simulink model "SingleInverterSim"  (R2020b)
settings: Solver=FixedStepAuto  StartTime=0.0  StopTime=3  FixedStep=Ts  RelTol=1e-3
values from neighbouring files (symbols this model uses):
  Cf = 0.02/W    (= 6.36619772368e-05)    [CalcSwingDroop.m]    (also in SingleInverterSim_Para.m = 0.02; SingleInverterSim_Para_v2.m = 0.02)
  Lc = 0.01/W    (= 3.18309886184e-05)    [CalcSwingDroop.m]    (also in SingleInverterSim_Para.m = 1e-09; SingleInverterSim_Para_v2.m = 0.01)
  Lf = 0.05/W    (= 0.000159154943092)    [CalcSwingDroop.m]    (also in SingleInverterSim_Para.m = 0.05; SingleInverterSim_Para_v2.m = 0.05)
  m = m*Wbase    (= 15.7079632679)    [CalcSwingDroop.m]    (also in SingleInverterSim_Para.m = 0.05; SingleInverterSim_Para_v2.m = 0.05)
  R_rated_GFL = X_rated_GFL/5    (= 0.08)    [SingleInverterSim_Para.m]
  R_rated_GFM = X_rated_GFM/5    (= 0.06)    [SingleInverterSim_Para.m]
  Sbase = 1    [MainAnalysisImpedanceCircuit.m]    (also in SingleInverterSim_Para.m; SingleInverterSim_Para_v2.m)
  Scale_ki_v = 20    [SingleInverterSim_Para.m]    (also in SingleInverterSim_Para_v2.m)
  Ts = 1/Fs    (= 0.0001)    [SingleInverterSim_Para.m]    (also in SingleInverterSim_Para_v2.m)
  Vbase = 1    [MainAnalysisImpedanceCircuit.m]    (also in SingleInverterSim_Para.m; SingleInverterSim_Para_v2.m)
  w_droop = 0.1*2*pi    (= 0.628318530718)    [SingleInverterSim_Para.m]    (also in SingleInverterSim_Para_v2.m = 62.8318530718)
  w_i_GFL = 250 *2*pi    (= 1570.79632679)    [SingleInverterSim_Para.m]    (also in SingleInverterSim_Para_v2.m = 3141.59265359)
  w_i_GFM = 500*2*pi    (= 3141.59265359)    [SingleInverterSim_Para.m]    (also in SingleInverterSim_Para_v2.m)
  w_pll = 15 *2*pi    (= 94.2477796077)    [SingleInverterSim_Para.m]    (also in SingleInverterSim_Para_v2.m = 62.8318530718)
  w_tau = 1e3 *2*pi    (= 6283.18530718)    [SingleInverterSim_Para.m]    (also in SingleInverterSim_Para_v2.m)
  w_v_GFM = 250 *2*pi    (= 1570.79632679)    [SingleInverterSim_Para.m]    (also in SingleInverterSim_Para_v2.m)
  Wbase = 2*pi*50    (= 314.159265359)    [CalcSwingDroop.m]    (also in MainAnalysisImpedanceCircuit.m; SingleInverterSim_Para.m; SingleInverterSim_Para_v2.m)
  X_rated_GFL = 0.4    [SingleInverterSim_Para.m]
  X_rated_GFM = 0.3    [SingleInverterSim_Para.m]
  Zbase = Vbase/Ibase    (= 1)    [MainAnalysisImpedanceCircuit.m]    (also in SingleInverterSim_Para.m; SingleInverterSim_Para_v2.m)
undefined symbols (not defined in the file or in its folder): DiscIntNeverNeededParam, initial, magnitude
libraries: powerlib x230, SimplexPS x57, SimplexPS_2015a x10, SimplusGT x3
(part 3 of 5)

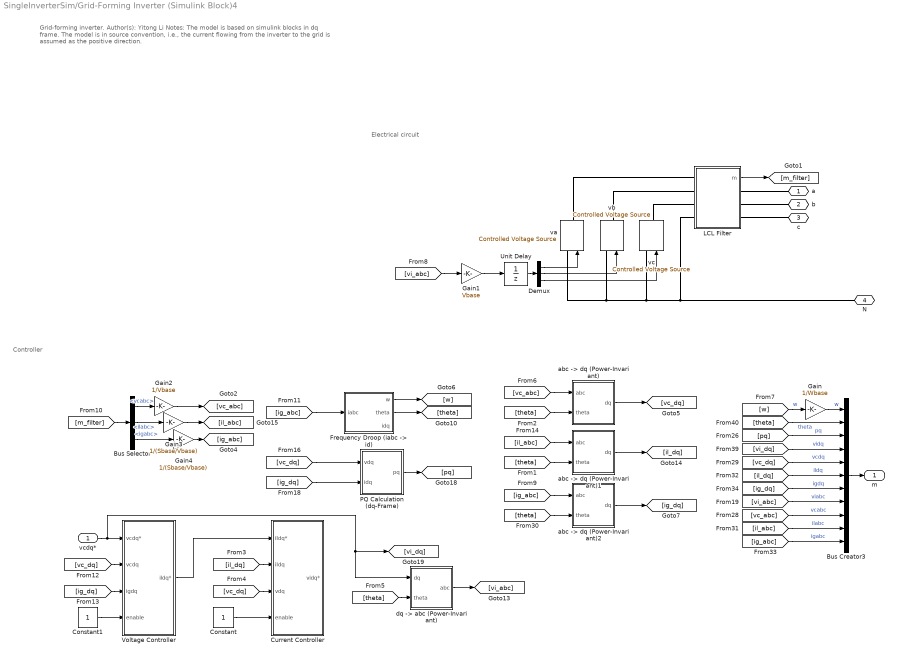
== system SingleInverterSim/Grid-Forming Inverter (Simulink Block)4 ==
  note: Grid-forming inverter.
      |
      | Author(s): Yitong Li
      |
      | Notes:
      |
      | The model is based on simulink blocks in dq frame.
      |
      | The model is in source convention, i.e., the current flowing from the inverter to the grid is assumed as the positive direction.
  note: Electrical circuit
  note: Controller
  vcdq* : Inport
  Bus Creator3 : BusCreator  Inputs=11
  Bus Selector : BusSelector  OutputSignals=vcabc,ilabc,igabc
  Constant : Constant
  Constant1 : Constant
  Current Controller : Subsystem  mask{Ts=Ts, Wbase=Wbase, Lf=Lf/Wbase, Kg=0, Kp=w_i*Lf/Wbase, Ki=w_i*w_i/4*Lf/Wbase, xdmax=inf, xqmax=inf, Kcd=0}
      mask prompts: Ts "Sampling Time (s)"; Wbase "Base Angular Frequency (rad/s)"; Lf "Inductance"; Kg "Estimator Gain"; Kp "Proportional Gain"; Ki "Integral Gain"; xdmax "Voltage D Limit"; xqmax "Voltage Q Limit"; Kcd "Cross Decoupling Gain"
  Demux : Demux  Outputs=3
  "Frequency Droop (iabc -> id)" : Subsystem  AncestorBlock=|  mask{Ts=Ts, Sbase=Sbase, Vbase=Vbase, Wbase=Wbase, m=m, w_tau=w_droop, theta0=0, i0=0, w0=1}
      | SimplusGT/Frequency Droop
      | (iabc -> id)
      mask prompts: Ts "Ts (s), samping period"; Sbase "Sbase (VA), base power"; Vbase "Vbase (V), base voltage"; Wbase "Wbase (rad/s), base angular frequency"; m "m (pu), droop gain"; w_tau "w_tau (rad/s), low-pass filter bandwidth"; theta0 "theta0 (rad), initial angle"; i0 "i0 (pu), current setting point"; w0 "w0 (pu), frequency setting point"
  Gain : Gain  Gain=1/Wbase
  Gain1 : Gain  Gain=Vbase
  Gain2 : Gain  Gain=1/Vbase
  Gain3 : Gain  Gain=1/(Sbase/Vbase)
  Gain4 : Gain  Gain=1/(Sbase/Vbase)
  LCL Filter : Subsystem  AncestorBlock=SimplexPS/LCL Filter  mask{Lf=Lf*(Vbase^2/Sbase)/Wbase, Rf=Lf*(Vbase^2/Sbase)/5, Lc=Lc*(Vbase^2/Sbase)/Wbase, Rc=Lc*(Vbase^2/Sbase)/5, Cf=Cf*(Sbase/Vbase^2)/Wbase, Rd=1e-5*(Vbase^2/Sbase)}
      mask prompts: Lf "Lf (H)"; Rf "Rf (Ohm)"; Lc "Lc (H)"; Rc "Rc (Ohm)"; Cf "Cf (F)"; Rd "Rd (Ohm)"
  PQ Calculation (dq-Frame) : Subsystem  AncestorBlock=|
      | SimplusGT/PQ Calculation
      | (dq-Frame)
  Unit Delay : UnitDelay  SampleTime=-1  HasFrameUpgradeWarning=on
  Voltage Controller : Subsystem  mask{Ts=Ts, Wbase=Wbase, Cf=Cf/Wbase, Kg=0, Kp=w_v*Cf/Wbase, Ki=w_v*w_v/4*Cf/Wbase*100, xdmax=inf, xqmax=inf, Kcd=0}
      mask prompts: Ts "Sampling Time (s)"; Wbase "Base Angular Frequency (rad/s)"; Cf "Capacitance"; Kg "Estimator Gain"; Kp "Proportional Gain"; Ki "Integral Gain"; xdmax "Current D Limit"; xqmax "Current Q Limit"; Kcd "Cross Decoupling Gain"
  "abc -> dq (Power-Invariant)" : Subsystem  AncestorBlock=|
      | SimplusGT/abc -> dq
      | (Power-Invariant)
  "abc -> dq (Power-Invariant)1" : Subsystem  AncestorBlock=|
      | SimplusGT/abc -> dq
      | (Power-Invariant)
  "abc -> dq (Power-Invariant)2" : Subsystem  AncestorBlock=|
      | SimplusGT/abc -> dq
      | (Power-Invariant)
  "dq -> abc (Power-Invariant)" : Subsystem  AncestorBlock=|
      | SimplusGT/dq -> abc
      | (Power-Invariant)
  va : powerlib/Electrical Sources/Controlled Voltage Source  Initialize=on  Source_Type=AC  Amplitude=0  Phase=0  Frequency=0  Measurements=None
  vb : powerlib/Electrical Sources/Controlled Voltage Source  Initialize=on  Source_Type=AC  Amplitude=0  Phase=0  Frequency=0  Measurements=None
  vc : powerlib/Electrical Sources/Controlled Voltage Source  Initialize=on  Source_Type=AC  Amplitude=0  Phase=0  Frequency=0  Measurements=None
  a : PMIOPort  Side=Right
  b : PMIOPort  Port=2  Side=Right
  c : PMIOPort  Port=3  Side=Right
  N : PMIOPort  Port=4  Side=Right
  m : Outport
  wires:
  Gain1/1 -> Unit Delay/1
  [vi_abc] -> Gain1/1
  Gain4/1 -> [ig_abc]
  Gain3/1 -> [il_abc]
  Gain2/1 -> [vc_abc]
  [ig_dq] -> Voltage Controller/3(igdq)
  [vc_dq] -> Voltage Controller/2(vcdq)
  Constant1/1 -> Voltage Controller/4(enable)
  Voltage Controller/1(ildq*) -> Current Controller/1(iIdq*)
  vcdq*/1 -> [vi_dq], "dq -> abc (Power-Invariant)"/1(dq), Voltage Controller/1(vcdq*)
  [ig_abc] -> Bus Creator3/11  "igabc"
  [il_abc] -> Bus Creator3/10  "ilabc"
  [vc_abc] -> Bus Creator3/9  "vcabc"
  [vi_abc] -> Bus Creator3/8  "viabc"
  [ig_dq] -> Bus Creator3/7  "igdq"
  [il_dq] -> Bus Creator3/6  "ildq"
  [vc_dq] -> Bus Creator3/5  "vcdq"
  [vi_dq] -> Bus Creator3/4  "vidq"
  [pq] -> Bus Creator3/3  "pq"
  [theta] -> Bus Creator3/2  "theta"
  Gain/1 -> Bus Creator3/1  "w"
  [w] -> Gain/1  "w"
  Bus Selector/1 -> Gain2/1  "<vcabc>"
  Unit Delay/1 -> Demux/1
  [m_filter] -> Bus Selector/1
  "abc -> dq (Power-Invariant)1"/1(dq) -> [il_dq]
  "abc -> dq (Power-Invariant)2"/1(dq) -> [ig_dq]
  "abc -> dq (Power-Invariant)"/1(dq) -> [vc_dq]
  [ig_abc] -> "Frequency Droop (iabc -> id)"/1(iabc)
  [il_dq] -> Current Controller/2(iIdq)
  [ig_dq] -> PQ Calculation (dq-Frame)/2(idq)
  PQ Calculation (dq-Frame)/1(pq) -> [pq]
  [vc_dq] -> PQ Calculation (dq-Frame)/1(vdq)
  [theta] -> "dq -> abc (Power-Invariant)"/2(theta)
  [vc_dq] -> Current Controller/3(vdq)
  Constant/1 -> Current Controller/4(enable)
  Bus Selector/2 -> Gain3/1  "<ilabc>"
  Bus Selector/3 -> Gain4/1  "<igabc>"
  [theta] -> "abc -> dq (Power-Invariant)2"/2(theta)
  [ig_abc] -> "abc -> dq (Power-Invariant)2"/1(abc)
  [il_abc] -> "abc -> dq (Power-Invariant)1"/1(abc)
  [vc_abc] -> "abc -> dq (Power-Invariant)"/1(abc)
  [theta] -> "abc -> dq (Power-Invariant)1"/2(theta)
  [theta] -> "abc -> dq (Power-Invariant)"/2(theta)
  Demux/3 -> vc/1
  Demux/2 -> vb/1
  Demux/1 -> va/1
  LCL Filter/1(m) -> [m_filter]
  Bus Creator3/1 -> m/1
  "dq -> abc (Power-Invariant)"/1(abc) -> [vi_abc]
  "Frequency Droop (iabc -> id)"/1(w) -> [w]
  "Frequency Droop (iabc -> id)"/2(theta) -> [theta]
  connections:
  LCL Filter/LConn3 -- vc/RConn1
  va/LConn1 -- vb/LConn1 -- vc/LConn1 -- LCL Filter/LConn4 -- N/RConn1
  LCL Filter/RConn3 -- c/RConn1
  LCL Filter/RConn2 -- b/RConn1
  LCL Filter/RConn1 -- a/RConn1
  LCL Filter/LConn1 -- va/RConn1
  LCL Filter/LConn2 -- vb/RConn1

== system SingleInverterSim/Grid-Following Inverter (Simulink Block)1/Current Controller ==
  iIdq* : Inport
  iIdq : Inport  Port=2
  vdq : Inport  Port=3
  enable : Inport  Port=4
  Constant : Constant  Value=Kcd
  Demux1 : Demux  Outputs=2
  Demux2 : Demux  Outputs=2
  Demux3 : Demux  Outputs=2
  Mux : Mux  Inputs=2
  PI-DT-Estimated d : Subsystem  mask{Lf=Lf, Kg=Kg, Kp=Kp, Ki=Ki, xmax=vdmax, xmin=-vdmax, Ts=Ts}
      mask prompts: Lf "Inductance"; Kg "Estimator Gain"; Kp "Proportional Gain"; Ki "Integral Gain"; xmax "Upper Limit"; xmin "Lower Limit"; Ts "Sampling Time"
  PI-DT-Estimated q : Subsystem  mask{Lf=Lf, Kg=Kg, Kp=Kp, Ki=Ki, xmax=vqmax, xmin=-vqmax, Ts=Ts}
      mask prompts: Lf "Inductance"; Kg "Estimator Gain"; Kp "Proportional Gain"; Ki "Integral Gain"; xmax "Upper Limit"; xmin "Lower Limit"; Ts "Sampling Time"
  Product : Product
  Product1 : Product
  sum_d : Sum  Inputs=+-
  sum_q : Sum
  wLd : Gain  Gain=Wbase*Lf
  wLq : Gain  Gain=Wbase*Lf
  vidq* : Outport
  wires:
  Constant/1 -> Product1/1, Product/2
  Product1/1 -> sum_d/2
  wLq/1 -> Product1/2
  Product/1 -> sum_q/1
  wLd/1 -> Product/1
  enable/1 -> PI-DT-Estimated d/1(enable), PI-DT-Estimated q/4(enable)
  Demux2/2 -> PI-DT-Estimated q/3(reference)
  Demux2/1 -> PI-DT-Estimated d/2(reference)
  iIdq*/1 -> Demux2/1
  Demux3/1 -> PI-DT-Estimated d/3(initial)
  Demux3/2 -> PI-DT-Estimated q/2(initial)
  PI-DT-Estimated q/1(Out) -> sum_q/2
  vdq/1 -> Demux3/1
  PI-DT-Estimated d/1(Out) -> sum_d/1
  Mux/1 -> vidq*/1
  Demux1/2 -> wLq/1, PI-DT-Estimated q/1(actual)
  Demux1/1 -> PI-DT-Estimated d/4(actual), wLd/1
  iIdq/1 -> Demux1/1
  sum_q/1 -> Mux/2
  sum_d/1 -> Mux/1

== system SingleInverterSim/Grid-Following Inverter (Simulink Block)1/LCL Filter ==
  note: Model for a LCL filter.
      |
      | Author(s): Yitong Li
      |
      | Notes:
      |
      | vi is the converter side voltage, and vg is the grid side voltage.
  Bus Creator : BusCreator  Inputs=5
  "LL -> LN1" : Subsystem  AncestorBlock=|
      | SimplusGT/Grid-Forming Inverter
      | (Simulink Block)/LCL Filter/LL -> LN1
  "LL -> LN2" : Subsystem  AncestorBlock=|
      | SimplusGT/Grid-Forming Inverter
      | (Simulink Block)/LCL Filter/LL -> LN1
  Mux{,1..4} (5 alike) : Mux  Inputs=3
  Three-Phase Series RLC Branch : powerlib/Elements/Three-Phase Series RLC Branch  LConnTagsString=A|B|C  RConnTagsString=A|B|C  BranchType=RL  Resistance=Rf  Inductance=Lf  Capacitance=1e-6  Measurements=None
  Three-Phase Series RLC Branch1 : powerlib/Elements/Three-Phase Series RLC Branch  LConnTagsString=A|B|C  RConnTagsString=A|B|C  BranchType=RL  Resistance=Rc  Inductance=Lc  Capacitance=1e-6  Measurements=None
  Three-Phase Series RLC Branch2 : powerlib/Elements/Three-Phase Series RLC Branch  LConnTagsString=A|B|C  RConnTagsString=A|B|C  BranchType=RC  Resistance=Rd  Inductance=Lc  Capacitance=Cf  Measurements=None
  Vab : powerlib/Measurements/Voltage Measurement  PhasorSimulation=off  OutputType=Complex  PSBequivalent=0
  Vab1 : powerlib/Measurements/Voltage Measurement  PhasorSimulation=off  OutputType=Complex  PSBequivalent=0
  Vbc : powerlib/Measurements/Voltage Measurement  PhasorSimulation=off  OutputType=Complex  PSBequivalent=0
  Vbc1 : powerlib/Measurements/Voltage Measurement  PhasorSimulation=off  OutputType=Complex  PSBequivalent=0
  Vca : powerlib/Measurements/Voltage Measurement  PhasorSimulation=off  OutputType=Complex  PSBequivalent=0
  Vca1 : powerlib/Measurements/Voltage Measurement  PhasorSimulation=off  OutputType=Complex  PSBequivalent=0
  iga : powerlib/Measurements/Current Measurement  PhasorSimulation=off  OutputType=Complex  PSBequivalent=0
  igb : powerlib/Measurements/Current Measurement  PhasorSimulation=off  OutputType=Complex  PSBequivalent=0
  igc : powerlib/Measurements/Current Measurement  PhasorSimulation=off  OutputType=Complex  PSBequivalent=0
  ila : powerlib/Measurements/Current Measurement  PhasorSimulation=off  OutputType=Complex  PSBequivalent=0
  ilb : powerlib/Measurements/Current Measurement  PhasorSimulation=off  OutputType=Complex  PSBequivalent=0
  ilc : powerlib/Measurements/Current Measurement  PhasorSimulation=off  OutputType=Complex  PSBequivalent=0
  vca measure : powerlib/Measurements/Voltage Measurement  PhasorSimulation=off  OutputType=Complex  PSBequivalent=0
  vcb measure : powerlib/Measurements/Voltage Measurement  PhasorSimulation=off  OutputType=Complex  PSBequivalent=0
  vcc measure : powerlib/Measurements/Voltage Measurement  PhasorSimulation=off  OutputType=Complex  PSBequivalent=0
  via : PMIOPort  Side=Left
  vib : PMIOPort  Port=2  Side=Left
  vic : PMIOPort  Port=3  Side=Left
  vga : PMIOPort  Port=4  Side=Right
  vgb : PMIOPort  Port=5  Side=Right
  vgc : PMIOPort  Port=6  Side=Right
  N : PMIOPort  Port=7  Side=Left
  m : Outport
  wires:
  Mux4/1 -> [igabc]
  ilb/1 -> Mux2/2
  ila/1 -> Mux2/1
  igc/1 -> Mux4/3
  vcc measure/1 -> Mux3/3
  Vab/1 -> Mux/1
  Mux/1 -> "LL -> LN1"/1(In1)
  vca measure/1 -> Mux3/1
  vcb measure/1 -> Mux3/2
  igb/1 -> Mux4/2
  iga/1 -> Mux4/1
  Vca/1 -> Mux/3
  ilc/1 -> Mux2/3
  Vbc/1 -> Mux/2
  Mux2/1 -> [ilabc]
  Bus Creator/1 -> m/1
  "LL -> LN1"/1(Out1) -> [vgabc]
  Mux3/1 -> [vcabc]
  Vbc1/1 -> Mux1/2
  Vca1/1 -> Mux1/3
  Mux1/1 -> "LL -> LN2"/1(In1)
  Vab1/1 -> Mux1/1
  "LL -> LN2"/1(Out1) -> [viabc]
  [viabc] -> Bus Creator/1  "viabc"
  [vcabc] -> Bus Creator/2  "vcabc"
  [vgabc] -> Bus Creator/3  "vgabc"
  [ilabc] -> Bus Creator/4  "ilabc"
  [igabc] -> Bus Creator/5  "igabc"
  connections:
  Three-Phase Series RLC Branch2/RConn1 -- Three-Phase Series RLC Branch2/RConn2 -- N/RConn1 -- Three-Phase Series RLC Branch2/RConn3 -- vcc measure/LConn2 -- vca measure/LConn2 -- vcb measure/LConn2
  Vca/LConn1 -- Vbc/LConn2 -- igc/RConn1 -- vgc/RConn1
  Vca1/LConn1 -- Vbc1/LConn2 -- vic/RConn1 -- Three-Phase Series RLC Branch/LConn3
  Three-Phase Series RLC Branch/LConn2 -- Vbc1/LConn1 -- Vab1/LConn2 -- vib/RConn1
  Vab1/LConn1 -- Vca1/LConn2 -- via/RConn1 -- Three-Phase Series RLC Branch/LConn1
  Three-Phase Series RLC Branch1/LConn3 -- ilc/RConn1 -- Three-Phase Series RLC Branch2/LConn3 -- vcc measure/LConn1
  Three-Phase Series RLC Branch1/RConn2 -- igb/LConn1
  Vbc/LConn1 -- Vab/LConn2 -- igb/RConn1 -- vgb/RConn1
  ilb/RConn1 -- Three-Phase Series RLC Branch1/LConn2 -- vcb measure/LConn1 -- Three-Phase Series RLC Branch2/LConn2
  ila/RConn1 -- Three-Phase Series RLC Branch1/LConn1 -- vca measure/LConn1 -- Three-Phase Series RLC Branch2/LConn1
  Vab/LConn1 -- Vca/LConn2 -- iga/RConn1 -- vga/RConn1
  Three-Phase Series RLC Branch1/RConn1 -- iga/LConn1
  Three-Phase Series RLC Branch1/RConn3 -- igc/LConn1
  Three-Phase Series RLC Branch/RConn1 -- ila/LConn1
  Three-Phase Series RLC Branch/RConn2 -- ilb/LConn1
  Three-Phase Series RLC Branch/RConn3 -- ilc/LConn1

== system SingleInverterSim/Grid-Following Inverter (Simulink Block)1/PLL (vabc -> vq) ==
  note: Measurement
  note: Gpll
  note: Phase lock loop (PLL)
      |
      | Author(s): Yitong Li
      |
      | Notes:
      |
      | vq is fed into the PI controller of the PLL.
  vabc : Inport
  Constant1 : Constant
  Constant2 : Constant  Value=theta0
  Constant3 : Constant
  Constant4 : Constant  Value=2*pi
  Constant6 : Constant  Value=0
  Demux1 : Demux  Outputs=2
  Discrete PI : Subsystem  AncestorBlock=SimplusGT/Discrete PI  mask{Kp=w_pll, Ki=w_pll*w_pll/4, xmax=inf, xmin=-inf, Ts=Ts}
      mask prompts: Kp "Proportional Gain"; Ki "Integral Gain"; xmax "Upper Limit"; xmin "Lower Limit"; Ts "Sampling Time"
  Discrete-Time Integrator : DiscreteIntegrator  SampleTime=Ts  ICPrevOutput=DiscIntNeverNeededParam  ICPrevScaledInput=DiscIntNeverNeededParam
  Filter p : DiscreteTransferFcn  Commented=on  Numerator=w_tau*Ts  Denominator=[1 ((w_tau*Ts)-1)]  SampleTime=Ts
  Gain1 : Gain  Gain=Wbase
  Gain4 : Gain  Gain=1/Wbase
  Gain5 : Gain  Gain=1/pi
  Math Function1 : Math  Operator=mod  SignedPower=on  SaturateOnIntegerOverflow=on
  Mux : Mux  Inputs=2
  Scope : Scope  NumInputPorts=4
  Sum : Sum
  Sum1 : Sum
  "abc -> dq (Power-Invariant)" : Subsystem  AncestorBlock=|
      | SimplusGT/abc -> dq
      | (Power-Invariant)
  w : Outport
  theta : Outport  Port=2
  vdq : Outport  Port=3
  wires:
  vabc/1 -> "abc -> dq (Power-Invariant)"/1(abc)
  "abc -> dq (Power-Invariant)"/1(dq) -> vdq/1, Demux1/1
  Constant4/1 -> Math Function1/2
  Constant6/1 -> Discrete PI/4(actual), Discrete PI/3(initial)
  Constant1/1 -> Discrete PI/1(enable)
  Discrete PI/1(Out) -> Sum/1
  Sum/1 -> [w], w/1, Discrete-Time Integrator/1
  Gain1/1 -> Sum/2
  Discrete-Time Integrator/1 -> Sum1/1
  Sum1/1 -> Math Function1/1
  Constant2/1 -> [theta0], Sum1/2
  Demux1/2 -> Discrete PI/2(reference), [vq]
  [vq] -> Scope/2  "vq"
  Mux/1 -> Gain5/1
  Gain4/1 -> Scope/3
  [w] -> Gain4/1  "w"
  [theta0] -> Mux/1  "theta0"
  [vd] -> Scope/1  "vd"
  Gain5/1 -> Scope/4
  [theta] -> Mux/2  "theta"
  Demux1/1 -> [vd]
  Constant3/1 -> Gain1/1
  Math Function1/1 -> "abc -> dq (Power-Invariant)"/2(theta), [theta], theta/1

== system SingleInverterSim/Grid-Following Inverter (Simulink Block)1/PQ Calculation (dq-Frame)1 ==
  note: Power calculation.
      |
      | Author(s): Yitong Li
      |
      | Notes:
      |
      | The calculation is done in dq frame.
  vdq : Inport
  idq : Inport  Port=2
  Mux : Mux  Inputs=2
  Mux1 : Mux  Inputs=2
  P = vd*id+vq*iq : Fcn  Expr=u[1]*u[3]+u[2]*u[4]
  Q = -vd*iq+vq*id : Fcn  Expr=-u[1]*u[4]+u[2]*u[3]
  pq : Outport
  wires:
  Mux/1 -> pq/1
  P = vd*id+vq*iq/1 -> Mux/1
  vdq/1 -> Mux1/1
  idq/1 -> Mux1/2
  Mux1/1 -> P = vd*id+vq*iq/1, Q = -vd*iq+vq*id/1
  Q = -vd*iq+vq*id/1 -> Mux/2

== system SingleInverterSim/Grid-Following Inverter (Simulink Block)1/abc -> dq (Power-Invariant)1 ==
  note: Frame transformation from abc to dq.
      |
      | Author(s): Yitong Li
      |
      | Notes:
      |
      | The transformation is power-invariant.
      |
      | theta is the angle that d axis leads a axis.
      |
      | q axis leads d axis by 90 degrees.
  abc : Inport
  theta : Inport  Port=2
  ->d : Fcn  Expr=cos(u(4))*u(1) + cos(u(4)-2/3*pi)*u(2) + cos(u(4)-4/3*pi)*u(3)
  ->q : Fcn  Expr=-sin(u(4))*u(1) - sin(u(4)-2/3*pi)*u(2) - sin(u(4)-4/3*pi)*u(3)
  Gain : Gain  Gain=sqrt(2/3)
  Mux5 : Mux  Inputs=2
  Mux6 : Mux  Inputs=2
  dq : Outport
  wires:
  abc/1 -> Gain/1
  ->d/1 -> Mux6/1
  Gain/1 -> Mux5/1
  theta/1 -> Mux5/2
  ->q/1 -> Mux6/2
  Mux6/1 -> dq/1
  Mux5/1 -> ->d/1, ->q/1

== system SingleInverterSim/Grid-Following Inverter (Simulink Block)1/abc -> dq (Power-Invariant)2 ==
  note: Frame transformation from abc to dq.
      |
      | Author(s): Yitong Li
      |
      | Notes:
      |
      | The transformation is power-invariant.
      |
      | theta is the angle that d axis leads a axis.
      |
      | q axis leads d axis by 90 degrees.
  abc : Inport
  theta : Inport  Port=2
  ->d : Fcn  Expr=cos(u(4))*u(1) + cos(u(4)-2/3*pi)*u(2) + cos(u(4)-4/3*pi)*u(3)
  ->q : Fcn  Expr=-sin(u(4))*u(1) - sin(u(4)-2/3*pi)*u(2) - sin(u(4)-4/3*pi)*u(3)
  Gain : Gain  Gain=sqrt(2/3)
  Mux5 : Mux  Inputs=2
  Mux6 : Mux  Inputs=2
  dq : Outport
  wires:
  abc/1 -> Gain/1
  ->d/1 -> Mux6/1
  Gain/1 -> Mux5/1
  theta/1 -> Mux5/2
  ->q/1 -> Mux6/2
  Mux6/1 -> dq/1
  Mux5/1 -> ->d/1, ->q/1

== system SingleInverterSim/Grid-Following Inverter (Simulink Block)1/abc -> dq (Power-Invariant)4 ==
  note: Frame transformation from abc to dq.
      |
      | Author(s): Yitong Li
      |
      | Notes:
      |
      | The transformation is power-invariant.
      |
      | theta is the angle that d axis leads a axis.
      |
      | q axis leads d axis by 90 degrees.
  abc : Inport
  theta : Inport  Port=2
  ->d : Fcn  Expr=cos(u(4))*u(1) + cos(u(4)-2/3*pi)*u(2) + cos(u(4)-4/3*pi)*u(3)
  ->q : Fcn  Expr=-sin(u(4))*u(1) - sin(u(4)-2/3*pi)*u(2) - sin(u(4)-4/3*pi)*u(3)
  Gain : Gain  Gain=sqrt(2/3)
  Mux5 : Mux  Inputs=2
  Mux6 : Mux  Inputs=2
  dq : Outport
  wires:
  abc/1 -> Gain/1
  ->d/1 -> Mux6/1
  Gain/1 -> Mux5/1
  theta/1 -> Mux5/2
  ->q/1 -> Mux6/2
  Mux6/1 -> dq/1
  Mux5/1 -> ->d/1, ->q/1

== system SingleInverterSim/Grid-Following Inverter (Simulink Block)1/dq -> abc (Power-Invariant)1 ==
  note: Frame transformation from dq to abc.
      |
      | Author(s): Yitong Li
      |
      | Notes:
      |
      | The transformation is power-invariant.
      |
      | theta is the angle that dq axis leads alpha/beta axis, specifically, d axis leads alpha axis.
  dq : Inport
  theta : Inport  Port=2
  ->a : Fcn  Expr=cos(u(3))*u(1) - sin(u(3))*u(2)
  ->b : Fcn  Expr=cos(u(3)-2/3*pi)*u(1) - sin(u(3)-2/3*pi)*u(2)
  ->c : Fcn  Expr=cos(u(3)-4/3*pi)*u(1) - sin(u(3)-4/3*pi)*u(2)
  Gain : Gain  Gain=sqrt(2/3)
  Mux5 : Mux  Inputs=2
  Mux6 : Mux  Inputs=3
  abc : Outport
  wires:
  ->b/1 -> Mux6/2
  ->a/1 -> Mux6/1
  Gain/1 -> Mux5/1
  dq/1 -> Gain/1
  ->c/1 -> Mux6/3
  Mux6/1 -> abc/1
  Mux5/1 -> ->b/1, ->a/1, ->c/1
  theta/1 -> Mux5/2

== system SingleInverterSim/Grid-Following Inverter (Simulink Block)2/Current Controller ==
  iIdq* : Inport
  iIdq : Inport  Port=2
  vdq : Inport  Port=3
  enable : Inport  Port=4
  Constant : Constant  Value=Kcd
  Demux1 : Demux  Outputs=2
  Demux2 : Demux  Outputs=2
  Demux3 : Demux  Outputs=2
  Mux : Mux  Inputs=2
  PI-DT-Estimated d : Subsystem  mask{Lf=Lf, Kg=Kg, Kp=Kp, Ki=Ki, xmax=vdmax, xmin=-vdmax, Ts=Ts}
      mask prompts: Lf "Inductance"; Kg "Estimator Gain"; Kp "Proportional Gain"; Ki "Integral Gain"; xmax "Upper Limit"; xmin "Lower Limit"; Ts "Sampling Time"
  PI-DT-Estimated q : Subsystem  mask{Lf=Lf, Kg=Kg, Kp=Kp, Ki=Ki, xmax=vqmax, xmin=-vqmax, Ts=Ts}
      mask prompts: Lf "Inductance"; Kg "Estimator Gain"; Kp "Proportional Gain"; Ki "Integral Gain"; xmax "Upper Limit"; xmin "Lower Limit"; Ts "Sampling Time"
  Product : Product
  Product1 : Product
  sum_d : Sum  Inputs=+-
  sum_q : Sum
  wLd : Gain  Gain=Wbase*Lf
  wLq : Gain  Gain=Wbase*Lf
  vidq* : Outport
  wires:
  sum_d/1 -> Mux/1
  sum_q/1 -> Mux/2
  iIdq/1 -> Demux1/1
  Demux1/1 -> wLd/1, PI-DT-Estimated d/4(actual)
  Demux1/2 -> PI-DT-Estimated q/1(actual), wLq/1
  Mux/1 -> vidq*/1
  PI-DT-Estimated d/1(Out) -> sum_d/1
  vdq/1 -> Demux3/1
  PI-DT-Estimated q/1(Out) -> sum_q/2
  Demux3/2 -> PI-DT-Estimated q/2(initial)
  Demux3/1 -> PI-DT-Estimated d/3(initial)
  iIdq*/1 -> Demux2/1
  Demux2/1 -> PI-DT-Estimated d/2(reference)
  Demux2/2 -> PI-DT-Estimated q/3(reference)
  enable/1 -> PI-DT-Estimated q/4(enable), PI-DT-Estimated d/1(enable)
  wLd/1 -> Product/1
  Product/1 -> sum_q/1
  wLq/1 -> Product1/2
  Product1/1 -> sum_d/2
  Constant/1 -> Product/2, Product1/1

== system SingleInverterSim/Grid-Following Inverter (Simulink Block)2/LCL Filter ==
  note: Model for a LCL filter.
      |
      | Author(s): Yitong Li
      |
      | Notes:
      |
      | vi is the converter side voltage, and vg is the grid side voltage.
  Bus Creator : BusCreator  Inputs=5
  "LL -> LN" : SimplexPS_2015a/LL -> LN  SystemSampleTime=-1  VariantActivationTime=update diagram  Latency=0  AutoFrameSizeCalculation=off
  "LL -> LN1" : SimplexPS_2015a/LL -> LN  SystemSampleTime=-1  VariantActivationTime=update diagram  Latency=0  AutoFrameSizeCalculation=off
  Mux{,1..4} (5 alike) : Mux  Inputs=3
  Three-Phase Series RLC Branch : powerlib/Elements/Three-Phase Series RLC Branch  LConnTagsString=A|B|C  RConnTagsString=A|B|C  BranchType=RL  Resistance=Rf  Inductance=Lf  Capacitance=1e-6  Measurements=None
  Three-Phase Series RLC Branch1 : powerlib/Elements/Three-Phase Series RLC Branch  LConnTagsString=A|B|C  RConnTagsString=A|B|C  BranchType=RL  Resistance=Rc  Inductance=Lc  Capacitance=1e-6  Measurements=None
  Three-Phase Series RLC Branch2 : powerlib/Elements/Three-Phase Series RLC Branch  LConnTagsString=A|B|C  RConnTagsString=A|B|C  BranchType=RC  Resistance=Rd  Inductance=Lc  Capacitance=Cf  Measurements=None
  Vab : powerlib/Measurements/Voltage Measurement  PhasorSimulation=off  OutputType=Complex  PSBequivalent=0
  Vab1 : powerlib/Measurements/Voltage Measurement  PhasorSimulation=off  OutputType=Complex  PSBequivalent=0
  Vbc : powerlib/Measurements/Voltage Measurement  PhasorSimulation=off  OutputType=Complex  PSBequivalent=0
  Vbc1 : powerlib/Measurements/Voltage Measurement  PhasorSimulation=off  OutputType=Complex  PSBequivalent=0
  Vca : powerlib/Measurements/Voltage Measurement  PhasorSimulation=off  OutputType=Complex  PSBequivalent=0
  Vca1 : powerlib/Measurements/Voltage Measurement  PhasorSimulation=off  OutputType=Complex  PSBequivalent=0
  iga : powerlib/Measurements/Current Measurement  PhasorSimulation=off  OutputType=Complex  PSBequivalent=0
  igb : powerlib/Measurements/Current Measurement  PhasorSimulation=off  OutputType=Complex  PSBequivalent=0
  igc : powerlib/Measurements/Current Measurement  PhasorSimulation=off  OutputType=Complex  PSBequivalent=0
  ila : powerlib/Measurements/Current Measurement  PhasorSimulation=off  OutputType=Complex  PSBequivalent=0
  ilb : powerlib/Measurements/Current Measurement  PhasorSimulation=off  OutputType=Complex  PSBequivalent=0
  ilc : powerlib/Measurements/Current Measurement  PhasorSimulation=off  OutputType=Complex  PSBequivalent=0
  vca measure : powerlib/Measurements/Voltage Measurement  PhasorSimulation=off  OutputType=Complex  PSBequivalent=0
  vcb measure : powerlib/Measurements/Voltage Measurement  PhasorSimulation=off  OutputType=Complex  PSBequivalent=0
  vcc measure : powerlib/Measurements/Voltage Measurement  PhasorSimulation=off  OutputType=Complex  PSBequivalent=0
  via : PMIOPort  Side=Left
  vib : PMIOPort  Port=2  Side=Left
  vic : PMIOPort  Port=3  Side=Left
  vga : PMIOPort  Port=4  Side=Right
  vgb : PMIOPort  Port=5  Side=Right
  vgc : PMIOPort  Port=6  Side=Right
  N : PMIOPort  Port=7  Side=Left
  m : Outport
  wires:
  [igabc] -> Bus Creator/5  "igabc"
  [ilabc] -> Bus Creator/4  "ilabc"
  [vgabc] -> Bus Creator/3  "vgabc"
  [vcabc] -> Bus Creator/2  "vcabc"
  [viabc] -> Bus Creator/1  "viabc"
  "LL -> LN"/1 -> [viabc]
  Vab1/1 -> Mux1/1
  Mux1/1 -> "LL -> LN"/1
  Vca1/1 -> Mux1/3
  Vbc1/1 -> Mux1/2
  Mux3/1 -> [vcabc]
  "LL -> LN1"/1 -> [vgabc]
  Bus Creator/1 -> m/1
  Mux2/1 -> [ilabc]
  Vbc/1 -> Mux/2
  ilc/1 -> Mux2/3
  Vca/1 -> Mux/3
  iga/1 -> Mux4/1
  igb/1 -> Mux4/2
  vcb measure/1 -> Mux3/2
  vca measure/1 -> Mux3/1
  Mux/1 -> "LL -> LN1"/1
  Vab/1 -> Mux/1
  vcc measure/1 -> Mux3/3
  igc/1 -> Mux4/3
  ila/1 -> Mux2/1
  ilb/1 -> Mux2/2
  Mux4/1 -> [igabc]
  connections:
  Three-Phase Series RLC Branch/RConn3 -- ilc/LConn1
  Three-Phase Series RLC Branch/RConn2 -- ilb/LConn1
  Three-Phase Series RLC Branch/RConn1 -- ila/LConn1
  Three-Phase Series RLC Branch1/RConn3 -- igc/LConn1
  Three-Phase Series RLC Branch1/RConn1 -- iga/LConn1
  vga/RConn1 -- iga/RConn1 -- Vca/LConn2 -- Vab/LConn1
  Three-Phase Series RLC Branch2/LConn1 -- vca measure/LConn1 -- Three-Phase Series RLC Branch1/LConn1 -- ila/RConn1
  Three-Phase Series RLC Branch2/LConn2 -- vcb measure/LConn1 -- Three-Phase Series RLC Branch1/LConn2 -- ilb/RConn1
  vgb/RConn1 -- igb/RConn1 -- Vab/LConn2 -- Vbc/LConn1
  Three-Phase Series RLC Branch1/RConn2 -- igb/LConn1
  vcc measure/LConn1 -- Three-Phase Series RLC Branch2/LConn3 -- ilc/RConn1 -- Three-Phase Series RLC Branch1/LConn3
  Three-Phase Series RLC Branch/LConn1 -- via/RConn1 -- Vca1/LConn2 -- Vab1/LConn1
  vib/RConn1 -- Vab1/LConn2 -- Vbc1/LConn1 -- Three-Phase Series RLC Branch/LConn2
  Three-Phase Series RLC Branch/LConn3 -- vic/RConn1 -- Vbc1/LConn2 -- Vca1/LConn1
  vgc/RConn1 -- igc/RConn1 -- Vbc/LConn2 -- Vca/LConn1
  vcb measure/LConn2 -- vca measure/LConn2 -- vcc measure/LConn2 -- Three-Phase Series RLC Branch2/RConn3 -- N/RConn1 -- Three-Phase Series RLC Branch2/RConn2 -- Three-Phase Series RLC Branch2/RConn1

== system SingleInverterSim/Grid-Following Inverter (Simulink Block)2/PLL (vabc -> vq) ==
  note: Phase lock loop (PLL)
      |
      | Author(s): Yitong Li
      |
      | Notes:
      |
      | vq is fed into the PI controller of the PLL.
  note: Gpll
  note: Measurement
  vabc : Inport
  Scale_PIpll : Inport  Port=2
  Constant1 : Constant
  Constant2 : Constant  Value=theta0
  Constant3 : Constant
  Constant4 : Constant  Value=2*pi
  Constant6 : Constant  Value=0
  Demux1 : Demux  Outputs=2
  Discrete PI : Subsystem  AncestorBlock=SimplexPS/Discrete PI  mask{Kp=w_pll, Ki=w_pll*w_pll/4, xmax=inf, xmin=-inf, Ts=Ts}
      mask prompts: Kp "Proportional Gain"; Ki "Integral Gain"; xmax "Upper Limit"; xmin "Lower Limit"; Ts "Sampling Time"
  Discrete-Time Integrator : DiscreteIntegrator  SampleTime=Ts  ICPrevOutput=DiscIntNeverNeededParam  ICPrevScaledInput=DiscIntNeverNeededParam
  Filter p : DiscreteTransferFcn  Numerator=w_tau*Ts  Denominator=[1 ((w_tau*Ts)-1)]  SampleTime=Ts
  Gain1 : Gain  Gain=Wbase
  Gain2 : Gain  Gain=1/Vbase
  Gain4 : Gain  Gain=1/Wbase
  Gain5 : Gain  Gain=1/pi
  Math Function1 : Math  Operator=mod  SignedPower=on  SaturateOnIntegerOverflow=on
  Mux : Mux  Inputs=2
  Scope : Scope  NumInputPorts=4
  Sum : Sum
  Sum1 : Sum
  "abc -> dq (Power-Invariant)" : SimplexPS/abc -> dq (Power-Invariant)  SystemSampleTime=-1  VariantActivationTime=update diagram  Latency=0  AutoFrameSizeCalculation=off
      settings: SourceProductName=Simplex Power Systems
  w : Outport
  theta : Outport  Port=2
  vdq : Outport  Port=3
  wires:
  Math Function1/1 -> theta/1, [theta], "abc -> dq (Power-Invariant)"/2
  Constant3/1 -> Gain1/1
  Demux1/1 -> [vd]
  [theta] -> Mux/2  "theta"
  Gain5/1 -> Scope/4
  [vd] -> Scope/1  "vd"
  [theta0] -> Mux/1  "theta0"
  [w] -> Gain4/1  "w"
  Gain4/1 -> Scope/3
  Mux/1 -> Gain5/1
  [vq] -> Scope/2  "vq"
  Filter p/1 -> Discrete PI/2(reference)
  Constant2/1 -> Sum1/2, [theta0]
  Sum1/1 -> Math Function1/1
  Discrete-Time Integrator/1 -> Sum1/1
  Gain1/1 -> Sum/2
  Sum/1 -> Discrete-Time Integrator/1, w/1, [w]
  Discrete PI/1(Out) -> Sum/1
  Constant1/1 -> Discrete PI/1(enable)
  Constant6/1 -> Discrete PI/3(initial), Discrete PI/4(actual)
  Demux1/2 -> Gain2/1, [vq]
  Gain2/1 -> Filter p/1
  Constant4/1 -> Math Function1/2
  "abc -> dq (Power-Invariant)"/1 -> Demux1/1, vdq/1
  vabc/1 -> "abc -> dq (Power-Invariant)"/1
  Scale_PIpll/1 -> Discrete PI/5(Scale_PIpll)

== system SingleInverterSim/Grid-Following Inverter (Simulink Block)3/Current Controller ==
  iIdq* : Inport
  iIdq : Inport  Port=2
  vdq : Inport  Port=3
  enable : Inport  Port=4
  Scale_PIi : Inport  Port=5
  Constant : Constant  Value=Kcd
  Demux1 : Demux  Outputs=2
  Demux2 : Demux  Outputs=2
  Demux3 : Demux  Outputs=2
  Mux : Mux  Inputs=2
  PI-DT-Estimated d : Subsystem  mask{Lf=Lf, Kg=Kg, Kp=Kp, Ki=Ki, xmax=vdmax, xmin=-vdmax, Ts=Ts}
      mask prompts: Lf "Inductance"; Kg "Estimator Gain"; Kp "Proportional Gain"; Ki "Integral Gain"; xmax "Upper Limit"; xmin "Lower Limit"; Ts "Sampling Time"
  PI-DT-Estimated q : Subsystem  mask{Lf=Lf, Kg=Kg, Kp=Kp, Ki=Ki, xmax=vqmax, xmin=-vqmax, Ts=Ts}
      mask prompts: Lf "Inductance"; Kg "Estimator Gain"; Kp "Proportional Gain"; Ki "Integral Gain"; xmax "Upper Limit"; xmin "Lower Limit"; Ts "Sampling Time"
  Product : Product
  Product1 : Product
  sum_d : Sum  Inputs=+-
  sum_q : Sum
  wLd : Gain  Gain=Wbase*Lf
  wLq : Gain  Gain=Wbase*Lf
  vidq* : Outport
  wires:
  sum_d/1 -> Mux/1
  sum_q/1 -> Mux/2
  iIdq/1 -> Demux1/1
  Demux1/1 -> wLd/1, PI-DT-Estimated d/4(actual)
  Demux1/2 -> PI-DT-Estimated q/1(actual), wLq/1
  Mux/1 -> vidq*/1
  PI-DT-Estimated d/1(Out) -> sum_d/1
  vdq/1 -> Demux3/1
  PI-DT-Estimated q/1(Out) -> sum_q/2
  Demux3/2 -> PI-DT-Estimated q/2(initial)
  Demux3/1 -> PI-DT-Estimated d/3(initial)
  iIdq*/1 -> Demux2/1
  Demux2/1 -> PI-DT-Estimated d/2(reference)
  Demux2/2 -> PI-DT-Estimated q/3(reference)
  enable/1 -> PI-DT-Estimated q/4(enable), PI-DT-Estimated d/1(enable)
  wLd/1 -> Product/1
  Product/1 -> sum_q/1
  wLq/1 -> Product1/2
  Product1/1 -> sum_d/2
  Constant/1 -> Product/2, Product1/1
  Scale_PIi/1 -> PI-DT-Estimated d/5(Scale_PIi), PI-DT-Estimated q/5(Scale_PIi)

== system SingleInverterSim/Grid-Following Inverter (Simulink Block)3/LCL Filter ==
  note: Model for a LCL filter.
      |
      | Author(s): Yitong Li
      |
      | Notes:
      |
      | vi is the converter side voltage, and vg is the grid side voltage.
  Bus Creator : BusCreator  Inputs=5
  "LL -> LN" : SimplexPS_2015a/LL -> LN  SystemSampleTime=-1  VariantActivationTime=update diagram  Latency=0  AutoFrameSizeCalculation=off
  "LL -> LN1" : SimplexPS_2015a/LL -> LN  SystemSampleTime=-1  VariantActivationTime=update diagram  Latency=0  AutoFrameSizeCalculation=off
  Mux{,1..4} (5 alike) : Mux  Inputs=3
  Three-Phase Series RLC Branch : powerlib/Elements/Three-Phase Series RLC Branch  LConnTagsString=A|B|C  RConnTagsString=A|B|C  BranchType=RL  Resistance=Rf  Inductance=Lf  Capacitance=1e-6  Measurements=None
  Three-Phase Series RLC Branch1 : powerlib/Elements/Three-Phase Series RLC Branch  LConnTagsString=A|B|C  RConnTagsString=A|B|C  BranchType=RL  Resistance=Rc  Inductance=Lc  Capacitance=1e-6  Measurements=None
  Three-Phase Series RLC Branch2 : powerlib/Elements/Three-Phase Series RLC Branch  LConnTagsString=A|B|C  RConnTagsString=A|B|C  BranchType=RC  Resistance=Rd  Inductance=Lc  Capacitance=Cf  Measurements=None
  Vab : powerlib/Measurements/Voltage Measurement  PhasorSimulation=off  OutputType=Complex  PSBequivalent=0
  Vab1 : powerlib/Measurements/Voltage Measurement  PhasorSimulation=off  OutputType=Complex  PSBequivalent=0
  Vbc : powerlib/Measurements/Voltage Measurement  PhasorSimulation=off  OutputType=Complex  PSBequivalent=0
  Vbc1 : powerlib/Measurements/Voltage Measurement  PhasorSimulation=off  OutputType=Complex  PSBequivalent=0
  Vca : powerlib/Measurements/Voltage Measurement  PhasorSimulation=off  OutputType=Complex  PSBequivalent=0
  Vca1 : powerlib/Measurements/Voltage Measurement  PhasorSimulation=off  OutputType=Complex  PSBequivalent=0
  iga : powerlib/Measurements/Current Measurement  PhasorSimulation=off  OutputType=Complex  PSBequivalent=0
  igb : powerlib/Measurements/Current Measurement  PhasorSimulation=off  OutputType=Complex  PSBequivalent=0
  igc : powerlib/Measurements/Current Measurement  PhasorSimulation=off  OutputType=Complex  PSBequivalent=0
  ila : powerlib/Measurements/Current Measurement  PhasorSimulation=off  OutputType=Complex  PSBequivalent=0
  ilb : powerlib/Measurements/Current Measurement  PhasorSimulation=off  OutputType=Complex  PSBequivalent=0
  ilc : powerlib/Measurements/Current Measurement  PhasorSimulation=off  OutputType=Complex  PSBequivalent=0
  vca measure : powerlib/Measurements/Voltage Measurement  PhasorSimulation=off  OutputType=Complex  PSBequivalent=0
  vcb measure : powerlib/Measurements/Voltage Measurement  PhasorSimulation=off  OutputType=Complex  PSBequivalent=0
  vcc measure : powerlib/Measurements/Voltage Measurement  PhasorSimulation=off  OutputType=Complex  PSBequivalent=0
  via : PMIOPort  Side=Left
  vib : PMIOPort  Port=2  Side=Left
  vic : PMIOPort  Port=3  Side=Left
  vga : PMIOPort  Port=4  Side=Right
  vgb : PMIOPort  Port=5  Side=Right
  vgc : PMIOPort  Port=6  Side=Right
  N : PMIOPort  Port=7  Side=Left
  m : Outport
  wires:
  [igabc] -> Bus Creator/5  "igabc"
  [ilabc] -> Bus Creator/4  "ilabc"
  [vgabc] -> Bus Creator/3  "vgabc"
  [vcabc] -> Bus Creator/2  "vcabc"
  [viabc] -> Bus Creator/1  "viabc"
  "LL -> LN"/1 -> [viabc]
  Vab1/1 -> Mux1/1
  Mux1/1 -> "LL -> LN"/1
  Vca1/1 -> Mux1/3
  Vbc1/1 -> Mux1/2
  Mux3/1 -> [vcabc]
  "LL -> LN1"/1 -> [vgabc]
  Bus Creator/1 -> m/1
  Mux2/1 -> [ilabc]
  Vbc/1 -> Mux/2
  ilc/1 -> Mux2/3
  Vca/1 -> Mux/3
  iga/1 -> Mux4/1
  igb/1 -> Mux4/2
  vcb measure/1 -> Mux3/2
  vca measure/1 -> Mux3/1
  Mux/1 -> "LL -> LN1"/1
  Vab/1 -> Mux/1
  vcc measure/1 -> Mux3/3
  igc/1 -> Mux4/3
  ila/1 -> Mux2/1
  ilb/1 -> Mux2/2
  Mux4/1 -> [igabc]
  connections:
  Three-Phase Series RLC Branch/RConn3 -- ilc/LConn1
  Three-Phase Series RLC Branch/RConn2 -- ilb/LConn1
  Three-Phase Series RLC Branch/RConn1 -- ila/LConn1
  Three-Phase Series RLC Branch1/RConn3 -- igc/LConn1
  Three-Phase Series RLC Branch1/RConn1 -- iga/LConn1
  vga/RConn1 -- iga/RConn1 -- Vca/LConn2 -- Vab/LConn1
  Three-Phase Series RLC Branch2/LConn1 -- vca measure/LConn1 -- Three-Phase Series RLC Branch1/LConn1 -- ila/RConn1
  Three-Phase Series RLC Branch2/LConn2 -- vcb measure/LConn1 -- Three-Phase Series RLC Branch1/LConn2 -- ilb/RConn1
  vgb/RConn1 -- igb/RConn1 -- Vab/LConn2 -- Vbc/LConn1
  Three-Phase Series RLC Branch1/RConn2 -- igb/LConn1
  vcc measure/LConn1 -- Three-Phase Series RLC Branch2/LConn3 -- ilc/RConn1 -- Three-Phase Series RLC Branch1/LConn3
  Three-Phase Series RLC Branch/LConn1 -- via/RConn1 -- Vca1/LConn2 -- Vab1/LConn1
  vib/RConn1 -- Vab1/LConn2 -- Vbc1/LConn1 -- Three-Phase Series RLC Branch/LConn2
  Three-Phase Series RLC Branch/LConn3 -- vic/RConn1 -- Vbc1/LConn2 -- Vca1/LConn1
  vgc/RConn1 -- igc/RConn1 -- Vbc/LConn2 -- Vca/LConn1
  vcb measure/LConn2 -- vca measure/LConn2 -- vcc measure/LConn2 -- Three-Phase Series RLC Branch2/RConn3 -- N/RConn1 -- Three-Phase Series RLC Branch2/RConn2 -- Three-Phase Series RLC Branch2/RConn1

== system SingleInverterSim/Grid-Forming Inverter (Simulink Block)/Current Controller ==
  iIdq* : Inport
  iIdq : Inport  Port=2
  vdq : Inport  Port=3
  enable : Inport  Port=4
  Constant : Constant  Value=Kcd
  Demux1 : Demux  Outputs=2
  Demux2 : Demux  Outputs=2
  Demux3 : Demux  Outputs=2
  Mux : Mux  Inputs=2
  PI-DT-Estimated d : Subsystem  mask{Lf=Lf, Kg=Kg, Kp=Kp, Ki=Ki, xmax=xdmax, xmin=-xdmax, Ts=Ts}
      mask prompts: Lf "Inductance"; Kg "Estimator Gain"; Kp "Proportional Gain"; Ki "Integral Gain"; xmax "Upper Limit"; xmin "Lower Limit"; Ts "Sampling Time"
  PI-DT-Estimated q : Subsystem  mask{Lf=Lf, Kg=Kg, Kp=Kp, Ki=Ki, xmax=xqmax, xmin=-xqmax, Ts=Ts}
      mask prompts: Lf "Inductance"; Kg "Estimator Gain"; Kp "Proportional Gain"; Ki "Integral Gain"; xmax "Upper Limit"; xmin "Lower Limit"; Ts "Sampling Time"
  Product : Product
  Product1 : Product
  sum_d : Sum  Inputs=+-
  sum_q : Sum
  wLd : Gain  Gain=Wbase*Lf
  wLq : Gain  Gain=Wbase*Lf
  vidq* : Outport
  wires:
  Constant/1 -> Product1/1, Product/2
  Product1/1 -> sum_d/2
  wLq/1 -> Product1/2
  Product/1 -> sum_q/1
  wLd/1 -> Product/1
  enable/1 -> PI-DT-Estimated d/1(enable), PI-DT-Estimated q/4(enable)
  Demux2/2 -> PI-DT-Estimated q/3(reference)
  Demux2/1 -> PI-DT-Estimated d/2(reference)
  iIdq*/1 -> Demux2/1
  Demux3/1 -> PI-DT-Estimated d/3(initial)
  Demux3/2 -> PI-DT-Estimated q/2(initial)
  PI-DT-Estimated q/1(Out) -> sum_q/2
  vdq/1 -> Demux3/1
  PI-DT-Estimated d/1(Out) -> sum_d/1
  Mux/1 -> vidq*/1
  Demux1/2 -> wLq/1, PI-DT-Estimated q/1(actual)
  Demux1/1 -> PI-DT-Estimated d/4(actual), wLd/1
  iIdq/1 -> Demux1/1
  sum_q/1 -> Mux/2
  sum_d/1 -> Mux/1

== system SingleInverterSim/Grid-Forming Inverter (Simulink Block)/Frequency Droop (iabc -> id) ==
  note: Measurement
  note: id-frequency droop controller
      |
      | Author(s): Yitong Li
      |
      | Notes:
      |
      | The current reference should be in source convention.
      |
      | It is a id-frequency droop controller rather than a power-frequency droop controller.
  iabc : Inport
  Constant : Constant  Value=w0
  Constant1 : Constant
  Constant2 : Constant  Value=theta0
  Constant4 : Constant  Value=2*pi
  Constant6 : Constant  Value=i0
  Demux1 : Demux  Outputs=2
  Discrete-Time Integrator : DiscreteIntegrator  SampleTime=Ts  ICPrevOutput=DiscIntNeverNeededParam  ICPrevScaledInput=DiscIntNeverNeededParam
  Filter p : DiscreteTransferFcn  Numerator=w_tau*Ts  Denominator=[1 ((w_tau*Ts)-1)]  SampleTime=Ts
  Gain2 : Gain  Gain=m
  Gain3 : Gain  Gain=Wbase
  Gain4 : Gain  Gain=1/Wbase
  Gain5 : Gain  Gain=1/pi
  Manual Switch : ManualSwitch
  Math Function1 : Math  Operator=mod  SignedPower=on  SaturateOnIntegerOverflow=on
  Mux : Mux  Inputs=2
  Scope : Scope  NumInputPorts=4
  Sum : Sum
  Sum1 : Sum
  Sum2 : Sum  Inputs=+-
  "abc -> dq (Power-Invariant)" : Subsystem  AncestorBlock=|
      | SimplusGT/abc -> dq
      | (Power-Invariant)
  w : Outport
  theta : Outport  Port=2
  idq : Outport  Port=3
  wires:
  Sum1/1 -> Math Function1/1
  Constant2/1 -> Sum1/2, [theta0]
  Math Function1/1 -> "abc -> dq (Power-Invariant)"/2(theta), [theta], theta/1
  Gain2/1 -> Sum/1
  Discrete-Time Integrator/1 -> Sum1/1
  Filter p/1 -> Sum2/2
  Constant/1 -> Sum/2
  "abc -> dq (Power-Invariant)"/1(dq) -> idq/1, Demux1/1
  Constant4/1 -> Math Function1/2
  iabc/1 -> "abc -> dq (Power-Invariant)"/1(abc)
  Constant6/1 -> Sum2/1
  Sum2/1 -> Gain2/1
  Gain3/1 -> [w], w/1, Discrete-Time Integrator/1
  Demux1/1 -> [id], Filter p/1  "id"
  Gain5/1 -> Scope/4
  [iq] -> Scope/2  "iq"
  [theta0] -> Mux/1  "theta"
  [id] -> Scope/1  "id"
  Mux/1 -> Gain5/1  "theta"
  [theta] -> Mux/2  "theta"
  Demux1/2 -> [iq]
  [w] -> Gain4/1  "w"
  Gain4/1 -> Scope/3
  Constant1/1 -> Manual Switch/2
  Sum/1 -> Manual Switch/1
  Manual Switch/1 -> Gain3/1

== system SingleInverterSim/Grid-Forming Inverter (Simulink Block)/LCL Filter ==
  note: Model for a LCL filter.
      |
      | Author(s): Yitong Li
      |
      | Notes:
      |
      | vi is the converter side voltage, and vg is the grid side voltage.
  Bus Creator : BusCreator  Inputs=5
  "LL -> LN" : Subsystem  AncestorBlock=SimplusGT/LL -> LN
  "LL -> LN1" : Subsystem  AncestorBlock=|
      | SimplusGT/Grid-Forming Inverter
      | (Simulink Block)/LCL Filter/LL -> LN
  Mux{,1..4} (5 alike) : Mux  Inputs=3
  Three-Phase Series RLC Branch : powerlib/Elements/Three-Phase Series RLC Branch  LConnTagsString=A|B|C  RConnTagsString=A|B|C  BranchType=RL  Resistance=Rf  Inductance=Lf  Capacitance=1e-6  Measurements=None
  Three-Phase Series RLC Branch1 : powerlib/Elements/Three-Phase Series RLC Branch  LConnTagsString=A|B|C  RConnTagsString=A|B|C  BranchType=RL  Resistance=Rc  Inductance=Lc  Capacitance=1e-6  Measurements=None
  Three-Phase Series RLC Branch2 : powerlib/Elements/Three-Phase Series RLC Branch  LConnTagsString=A|B|C  RConnTagsString=A|B|C  BranchType=RC  Resistance=Rd  Inductance=Lc  Capacitance=Cf  Measurements=None
  Vab : powerlib/Measurements/Voltage Measurement  PhasorSimulation=off  OutputType=Complex  PSBequivalent=0
  Vab1 : powerlib/Measurements/Voltage Measurement  PhasorSimulation=off  OutputType=Complex  PSBequivalent=0
  Vbc : powerlib/Measurements/Voltage Measurement  PhasorSimulation=off  OutputType=Complex  PSBequivalent=0
  Vbc1 : powerlib/Measurements/Voltage Measurement  PhasorSimulation=off  OutputType=Complex  PSBequivalent=0
  Vca : powerlib/Measurements/Voltage Measurement  PhasorSimulation=off  OutputType=Complex  PSBequivalent=0
  Vca1 : powerlib/Measurements/Voltage Measurement  PhasorSimulation=off  OutputType=Complex  PSBequivalent=0
  iga : powerlib/Measurements/Current Measurement  PhasorSimulation=off  OutputType=Complex  PSBequivalent=0
  igb : powerlib/Measurements/Current Measurement  PhasorSimulation=off  OutputType=Complex  PSBequivalent=0
  igc : powerlib/Measurements/Current Measurement  PhasorSimulation=off  OutputType=Complex  PSBequivalent=0
  ila : powerlib/Measurements/Current Measurement  PhasorSimulation=off  OutputType=Complex  PSBequivalent=0
  ilb : powerlib/Measurements/Current Measurement  PhasorSimulation=off  OutputType=Complex  PSBequivalent=0
  ilc : powerlib/Measurements/Current Measurement  PhasorSimulation=off  OutputType=Complex  PSBequivalent=0
  vca measure : powerlib/Measurements/Voltage Measurement  PhasorSimulation=off  OutputType=Complex  PSBequivalent=0
  vcb measure : powerlib/Measurements/Voltage Measurement  PhasorSimulation=off  OutputType=Complex  PSBequivalent=0
  vcc measure : powerlib/Measurements/Voltage Measurement  PhasorSimulation=off  OutputType=Complex  PSBequivalent=0
  via : PMIOPort  Side=Left
  vib : PMIOPort  Port=2  Side=Left
  vic : PMIOPort  Port=3  Side=Left
  vga : PMIOPort  Port=4  Side=Right
  vgb : PMIOPort  Port=5  Side=Right
  vgc : PMIOPort  Port=6  Side=Right
  N : PMIOPort  Port=7  Side=Left
  m : Outport
  wires:
  Mux4/1 -> [igabc]
  ilb/1 -> Mux2/2
  ila/1 -> Mux2/1
  igc/1 -> Mux4/3
  vcc measure/1 -> Mux3/3
  Vab/1 -> Mux/1
  Mux/1 -> "LL -> LN1"/1(In1)
  vca measure/1 -> Mux3/1
  vcb measure/1 -> Mux3/2
  igb/1 -> Mux4/2
  iga/1 -> Mux4/1
  Vca/1 -> Mux/3
  ilc/1 -> Mux2/3
  Vbc/1 -> Mux/2
  Mux2/1 -> [ilabc]
  Bus Creator/1 -> m/1
  "LL -> LN1"/1(Out1) -> [vgabc]
  Mux3/1 -> [vcabc]
  Vbc1/1 -> Mux1/2
  Vca1/1 -> Mux1/3
  Mux1/1 -> "LL -> LN"/1(In1)
  Vab1/1 -> Mux1/1
  "LL -> LN"/1(Out1) -> [viabc]
  [viabc] -> Bus Creator/1  "viabc"
  [vcabc] -> Bus Creator/2  "vcabc"
  [vgabc] -> Bus Creator/3  "vgabc"
  [ilabc] -> Bus Creator/4  "ilabc"
  [igabc] -> Bus Creator/5  "igabc"
  connections:
  Three-Phase Series RLC Branch2/RConn1 -- Three-Phase Series RLC Branch2/RConn2 -- N/RConn1 -- Three-Phase Series RLC Branch2/RConn3 -- vcc measure/LConn2 -- vca measure/LConn2 -- vcb measure/LConn2
  Vca/LConn1 -- Vbc/LConn2 -- igc/RConn1 -- vgc/RConn1
  Vca1/LConn1 -- Vbc1/LConn2 -- vic/RConn1 -- Three-Phase Series RLC Branch/LConn3
  Three-Phase Series RLC Branch/LConn2 -- Vbc1/LConn1 -- Vab1/LConn2 -- vib/RConn1
  Vab1/LConn1 -- Vca1/LConn2 -- via/RConn1 -- Three-Phase Series RLC Branch/LConn1
  Three-Phase Series RLC Branch1/LConn3 -- ilc/RConn1 -- Three-Phase Series RLC Branch2/LConn3 -- vcc measure/LConn1
  Three-Phase Series RLC Branch1/RConn2 -- igb/LConn1
  Vbc/LConn1 -- Vab/LConn2 -- igb/RConn1 -- vgb/RConn1
  ilb/RConn1 -- Three-Phase Series RLC Branch1/LConn2 -- vcb measure/LConn1 -- Three-Phase Series RLC Branch2/LConn2
  ila/RConn1 -- Three-Phase Series RLC Branch1/LConn1 -- vca measure/LConn1 -- Three-Phase Series RLC Branch2/LConn1
  Vab/LConn1 -- Vca/LConn2 -- iga/RConn1 -- vga/RConn1
  Three-Phase Series RLC Branch1/RConn1 -- iga/LConn1
  Three-Phase Series RLC Branch1/RConn3 -- igc/LConn1
  Three-Phase Series RLC Branch/RConn1 -- ila/LConn1
  Three-Phase Series RLC Branch/RConn2 -- ilb/LConn1
  Three-Phase Series RLC Branch/RConn3 -- ilc/LConn1

== system SingleInverterSim/Grid-Forming Inverter (Simulink Block)/PQ Calculation (dq-Frame) ==
  note: Power calculation.
      |
      | Author(s): Yitong Li
      |
      | Notes:
      |
      | The calculation is done in dq frame.
  vdq : Inport
  idq : Inport  Port=2
  Mux : Mux  Inputs=2
  Mux1 : Mux  Inputs=2
  P = vd*id+vq*iq : Fcn  Expr=u[1]*u[3]+u[2]*u[4]
  Q = -vd*iq+vq*id : Fcn  Expr=-u[1]*u[4]+u[2]*u[3]
  pq : Outport
  wires:
  Q = -vd*iq+vq*id/1 -> Mux/2
  Mux1/1 -> Q = -vd*iq+vq*id/1, P = vd*id+vq*iq/1
  idq/1 -> Mux1/2
  vdq/1 -> Mux1/1
  P = vd*id+vq*iq/1 -> Mux/1
  Mux/1 -> pq/1

== system SingleInverterSim/Grid-Forming Inverter (Simulink Block)/Voltage Controller ==
  vcdq* : Inport
  vcdq : Inport  Port=2
  igdq : Inport  Port=3
  enable : Inport  Port=4
  Constant : Constant  Value=Kcd
  Demux1 : Demux  Outputs=2
  Demux2 : Demux  Outputs=2
  Demux3 : Demux  Outputs=2
  Mux : Mux  Inputs=2
  PI-DT-Estimated d : Subsystem  mask{Kg=Kg, Kp=Kp, Ki=Ki, xmax=xdmax, xmin=-xdmax, Ts=Ts}
      mask prompts: Kg "Estimator Gain"; Kp "Proportional Gain"; Ki "Integral Gain"; xmax "Upper Limit"; xmin "Lower Limit"; Ts "Sampling Time"
  PI-DT-Estimated q : Subsystem  mask{Kg=Kg, Kp=Kp, Ki=Ki, xmax=xqmax, xmin=-xqmax, Ts=Ts}
      mask prompts: Kg "Estimator Gain"; Kp "Proportional Gain"; Ki "Integral Gain"; xmax "Upper Limit"; xmin "Lower Limit"; Ts "Sampling Time"
  Product : Product
  Product1 : Product
  sum_d : Sum  Inputs=+-
  sum_q : Sum
  wCd : Gain  Gain=Wbase*Cf
  wCq : Gain  Gain=Wbase*Cf
  ildq* : Outport
  wires:
  Constant/1 -> Product1/1, Product/2
  Product1/1 -> sum_d/2
  wCq/1 -> Product1/2
  Product/1 -> sum_q/1
  wCd/1 -> Product/1
  enable/1 -> PI-DT-Estimated d/1(enable), PI-DT-Estimated q/4(enable)
  Demux2/2 -> PI-DT-Estimated q/3(reference)
  Demux2/1 -> PI-DT-Estimated d/2(reference)
  vcdq*/1 -> Demux2/1
  Demux3/1 -> PI-DT-Estimated d/3(initial)
  Demux3/2 -> PI-DT-Estimated q/2(initial)
  PI-DT-Estimated q/1(Out) -> sum_q/2
  igdq/1 -> Demux3/1
  PI-DT-Estimated d/1(Out) -> sum_d/1
  Mux/1 -> ildq*/1
  Demux1/2 -> wCq/1, PI-DT-Estimated q/1(actual)
  Demux1/1 -> PI-DT-Estimated d/4(actual), wCd/1
  vcdq/1 -> Demux1/1
  sum_q/1 -> Mux/2
  sum_d/1 -> Mux/1

== system SingleInverterSim/Grid-Forming Inverter (Simulink Block)/abc -> dq (Power-Invariant) ==
  note: Frame transformation from abc to dq.
      |
      | Author(s): Yitong Li
      |
      | Notes:
      |
      | The transformation is power-invariant.
      |
      | theta is the angle that d axis leads a axis.
      |
      | q axis leads d axis by 90 degrees.
  abc : Inport
  theta : Inport  Port=2
  ->d : Fcn  Expr=cos(u(4))*u(1) + cos(u(4)-2/3*pi)*u(2) + cos(u(4)-4/3*pi)*u(3)
  ->q : Fcn  Expr=-sin(u(4))*u(1) - sin(u(4)-2/3*pi)*u(2) - sin(u(4)-4/3*pi)*u(3)
  Gain : Gain  Gain=sqrt(2/3)
  Mux5 : Mux  Inputs=2
  Mux6 : Mux  Inputs=2
  dq : Outport
  wires:
  Mux5/1 -> ->q/1, ->d/1
  Mux6/1 -> dq/1
  ->q/1 -> Mux6/2
  theta/1 -> Mux5/2
  Gain/1 -> Mux5/1
  ->d/1 -> Mux6/1
  abc/1 -> Gain/1

== system SingleInverterSim/Grid-Forming Inverter (Simulink Block)/abc -> dq (Power-Invariant)1 ==
  note: Frame transformation from abc to dq.
      |
      | Author(s): Yitong Li
      |
      | Notes:
      |
      | The transformation is power-invariant.
      |
      | theta is the angle that d axis leads a axis.
      |
      | q axis leads d axis by 90 degrees.
  abc : Inport
  theta : Inport  Port=2
  ->d : Fcn  Expr=cos(u(4))*u(1) + cos(u(4)-2/3*pi)*u(2) + cos(u(4)-4/3*pi)*u(3)
  ->q : Fcn  Expr=-sin(u(4))*u(1) - sin(u(4)-2/3*pi)*u(2) - sin(u(4)-4/3*pi)*u(3)
  Gain : Gain  Gain=sqrt(2/3)
  Mux5 : Mux  Inputs=2
  Mux6 : Mux  Inputs=2
  dq : Outport
  wires:
  Mux5/1 -> ->q/1, ->d/1
  Mux6/1 -> dq/1
  ->q/1 -> Mux6/2
  theta/1 -> Mux5/2
  Gain/1 -> Mux5/1
  ->d/1 -> Mux6/1
  abc/1 -> Gain/1
